simulink model "v_koordynacja"  (R2015a)
settings: Solver=ode45  StartTime=0.0  StopTime=20  RelTol=1e-3
settings Model: Creator=Marta  LastModifiedBy=Marta

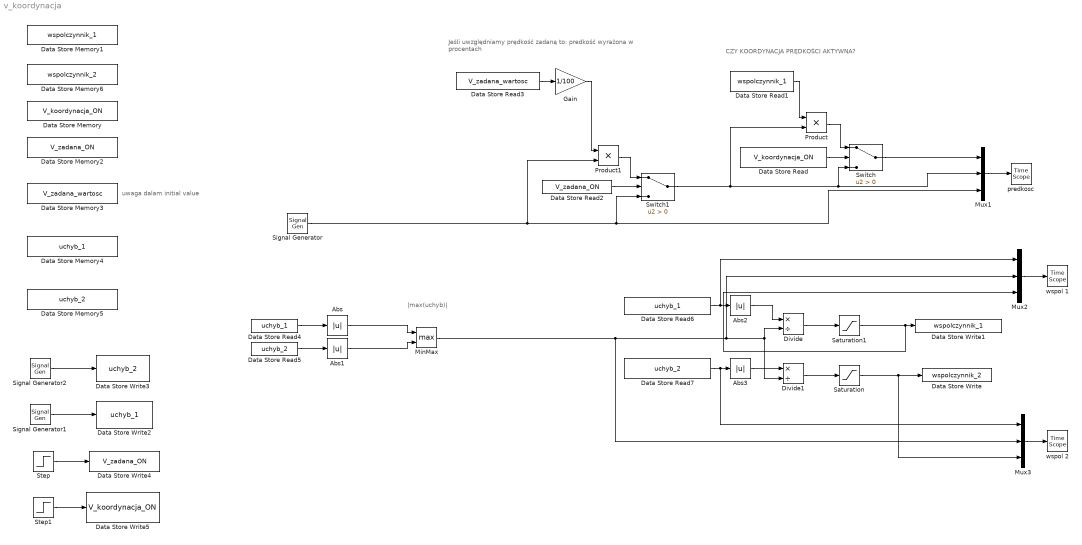
== system v_koordynacja ==
  note: uwaga dalam initial value
  note: |max(uchyb)|
  note: CZY KOORDYNACJA PRĘDKOŚCI AKTYWNA?
  note: Jeśli uwzględniamy prędkość zadaną to: predkość wyrażona w procentach
  Abs{,1..3} (4 alike) : Abs
  Data Store Memory : DataStoreMemory  DataStoreName=V_koordynacja_ON  ReadBeforeWriteMsg=warning  WriteAfterWriteMsg=warning  WriteAfterReadMsg=warning
  Data Store Memory1 : DataStoreMemory  DataStoreName=wspolczynnik_1  ReadBeforeWriteMsg=warning  WriteAfterWriteMsg=warning  WriteAfterReadMsg=warning
  Data Store Memory2 : DataStoreMemory  DataStoreName=V_zadana_ON  ReadBeforeWriteMsg=warning  WriteAfterWriteMsg=warning  WriteAfterReadMsg=warning
  Data Store Memory3 : DataStoreMemory  DataStoreName=V_zadana_wartosc  ReadBeforeWriteMsg=warning  WriteAfterWriteMsg=warning  WriteAfterReadMsg=warning  InitialValue=50
  Data Store Memory4 : DataStoreMemory  DataStoreName=uchyb_1  ReadBeforeWriteMsg=warning  WriteAfterWriteMsg=warning  WriteAfterReadMsg=warning
  Data Store Memory5 : DataStoreMemory  DataStoreName=uchyb_2  ReadBeforeWriteMsg=warning  WriteAfterWriteMsg=warning  WriteAfterReadMsg=warning
  Data Store Memory6 : DataStoreMemory  DataStoreName=wspolczynnik_2  ReadBeforeWriteMsg=warning  WriteAfterWriteMsg=warning  WriteAfterReadMsg=warning
  Data Store Read : DataStoreRead  DataStoreName=V_koordynacja_ON
  Data Store Read1 : DataStoreRead  DataStoreName=wspolczynnik_1
  Data Store Read2 : DataStoreRead  DataStoreName=V_zadana_ON
  Data Store Read3 : DataStoreRead  DataStoreName=V_zadana_wartosc
  Data Store Read4 : DataStoreRead  DataStoreName=uchyb_1
  Data Store Read5 : DataStoreRead  DataStoreName=uchyb_2
  Data Store Read6 : DataStoreRead  DataStoreName=uchyb_1
  Data Store Read7 : DataStoreRead  DataStoreName=uchyb_2
  Data Store Write : DataStoreWrite  DataStoreName=wspolczynnik_2
  Data Store Write1 : DataStoreWrite  DataStoreName=wspolczynnik_1
  Data Store Write2 : DataStoreWrite  DataStoreName=uchyb_1
  Data Store Write3 : DataStoreWrite  DataStoreName=uchyb_2
  Data Store Write4 : DataStoreWrite  DataStoreName=V_zadana_ON
  Data Store Write5 : DataStoreWrite  DataStoreName=V_koordynacja_ON
  Divide : Product  Inputs=*/
  Divide1 : Product  Inputs=*/
  Gain : Gain  Gain=1/100
  MinMax : MinMax  Function=max  Inputs=2
  Mux1 : Mux  Inputs=3
  Mux2 : Mux  Inputs=3
  Mux3 : Mux  Inputs=3
  Product : Product
  Product1 : Product
  Saturation : Saturate  UpperLimit=1  LowerLimit=0.05
  Saturation1 : Saturate  UpperLimit=1  LowerLimit=0.05
  Signal Generator : SignalGenerator  Units=rad/sec
  Signal Generator1 : SignalGenerator  Amplitude=5  Frequency=2  Units=rad/sec
  Signal Generator2 : SignalGenerator  Amplitude=5  Units=rad/sec
  Step : Step  Time=2  SampleTime=0
  Step1 : Step  Time=5  SampleTime=0
  Switch : Switch  Criteria=u2 > Threshold
  Switch1 : Switch  Criteria=u2 > Threshold
  "predkosc " : TimeScope
  "wspol 1 " : TimeScope
  "wspol 2 " : TimeScope
  wires:
  Data Store Read/1 -> Switch/2
  Product/1 -> Switch/1
  Data Store Read1/1 -> Product/1
  Data Store Read2/1 -> Switch1/2
  Product1/1 -> Switch1/1
  Data Store Read3/1 -> Gain/1
  Gain/1 -> Product1/1
  Data Store Read5/1 -> Abs1/1
  Data Store Read4/1 -> Abs/1
  Abs/1 -> MinMax/1
  Abs1/1 -> MinMax/2
  Data Store Read6/1 -> Mux2/1, Abs2/1
  Data Store Read7/1 -> Mux3/1, Abs3/1
  Divide1/1 -> Saturation/1
  Saturation/1 -> Mux3/3, Data Store Write/1
  Divide/1 -> Saturation1/1
  Saturation1/1 -> Mux2/3, Data Store Write1/1
  Abs2/1 -> Divide/1
  Abs3/1 -> Divide1/1
  MinMax/1 -> Mux3/2, Mux2/2, Divide/2, Divide1/2
  Signal Generator1/1 -> Data Store Write2/1
  Signal Generator2/1 -> Data Store Write3/1
  Step/1 -> Data Store Write4/1
  Step1/1 -> Data Store Write5/1
  Switch/1 -> Mux1/1
  Mux2/1 -> "wspol 1 "/1
  Mux3/1 -> "wspol 2 "/1
  Switch1/1 -> Product/2, Mux1/2, Switch/3
  Signal Generator/1 -> Mux1/3, Switch1/3, Product1/2
  Mux1/1 -> "predkosc "/1
